simulink model "index_simulink"  (R2024b)
settings: Solver=FixedStepAuto  StartTime=0.0  StopTime=1000.0  FixedStep=0.001  RelTol=1e-3
libraries: root x1
settings Model: Creator=mainuser  LastModifiedBy=mainuser

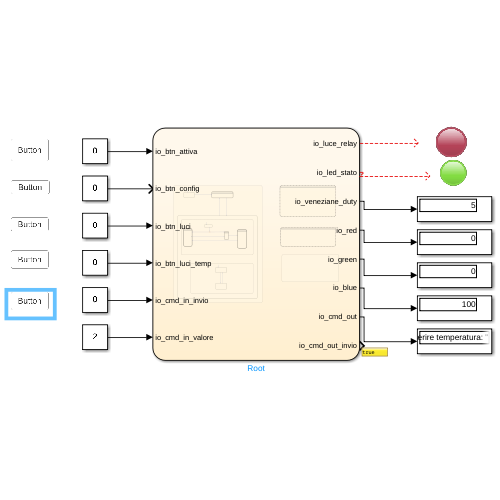
[thumbnail: Simulink's stored preview of the top-level diagram]
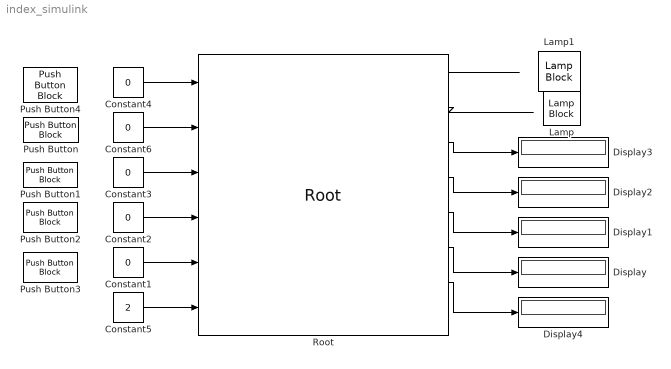
== system index_simulink ==
  Constant{1..4,6} (5 alike) : Constant  Value=0  OutDataTypeStr=boolean
  Constant5 : Constant  Value=2  OutDataTypeStr=uint8
  Display{,1..4} (5 alike) : Display
  Lamp : LampBlock  LabelPosition=Hide
  Lamp1 : LampBlock  LabelPosition=Hide
  Push Button{,1..4} (5 alike) : PushButtonBlock  OffValue=0.000000
  Root : root/Root  SystemSampleTime=-1  VariantActivationTime=update diagram  AllowFlexibleInterface=on  Latency=0  AutoFrameSizeCalculation=off
  wires:
  Constant6/1 -> Root/2
  Constant3/1 -> Root/3
  Constant2/1 -> Root/4
  Constant1/1 -> Root/5
  Constant4/1 -> Root/1
  Constant5/1 -> Root/6
  Root/6 -> Display/1
  Root/5 -> Display1/1
  Root/4 -> Display2/1
  Root/3 -> Display3/1
  Root/7 -> Display4/1
  Root/2 -> ?
  Root/1 -> ?
